simulink subsystem "NIBP_NoiseRemovalFilter_SR"  (R2021b)
settings: Solver=VariableStepAuto  StartTime=0.0  StopTime=10.0  RelTol=1e-3
libraries: Heart_Signal_Processing_Library x5
settings Model: Creator=wallyproenza  LastModifiedBy=wallyproenza

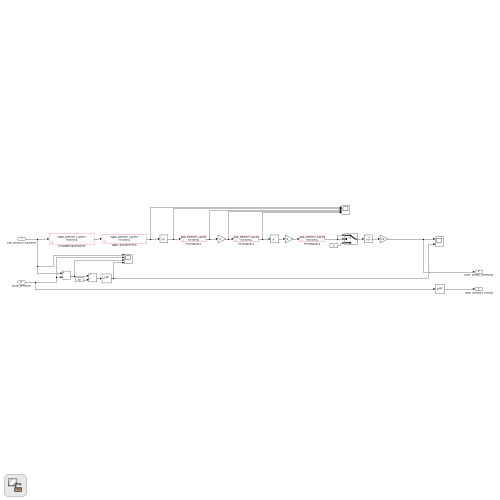
[thumbnail: Simulink's stored preview of the top-level diagram]
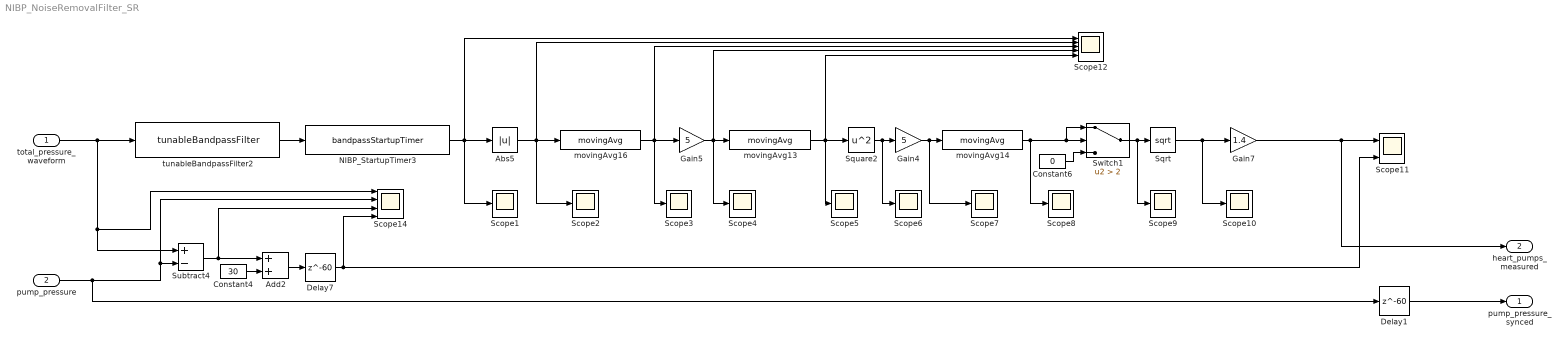
== system NIBP_NoiseRemovalFilter_SR ==
  total_pressure_waveform : Inport
  pump_pressure : Inport  Port=2
  Abs5 : Abs
  Add2 : Sum
  Constant4 : Constant  Value=30
  Constant6 : Constant  Value=0
  Delay1 : Delay  DelayLength=60  InitialCondition=0
  Delay7 : Delay  DelayLength=60  InitialCondition=0
  Gain4 : Gain  Gain=5
  Gain5 : Gain  Gain=5
  Gain7 : Gain  Gain=1.4
  NIBP_StartupTimer3 : Heart_Signal_Processing_Library/bandpassStartupTimer  Description=|  SystemSampleTime=-1  VariantActivationTime=update diagram  Latency=0  AutoFrameSizeCalculation=off
      | The bandpassStartupTimer acts as a temporary buffer between the first 0.5 seconds of the chosen bandpass and the derivative filters.
      | Outputs 0 prior to the 0.5 seconds, and then passes the bandpass filter otuput into the derivative filter after the 0.5 seconds. This component 
      | helps eliminate the possiblility of false negatives caused by an abnormally high signal threshold initial values that could occur prior to 0.5 seconds.
  Scope{1..10} (10 alike) : Scope
  Scope11 : Scope  NumInputPorts=2
  Scope12 : Scope  NumInputPorts=5
  Scope14 : Scope  NumInputPorts=4
  Sqrt : Sqrt  SaturateOnIntegerOverflow=on
  Square2 : Math  Operator=square  SaturateOnIntegerOverflow=on
  Subtract4 : Sum  Inputs=+-
  Switch1 : Switch  Criteria=u2 > Threshold  Threshold=2
  movingAvg13 : Heart_Signal_Processing_Library/movingAvg  Description=|  SystemSampleTime=-1  VariantActivationTime=update diagram  Latency=0  AutoFrameSizeCalculation=off
      | The movingAvg (moving average) filter is designed to be placed after a squaring function (which should have been placed right after the derivative filter),
      | and is a done so that the area where the QRS is present is expanded in regards to timespan. 
      | 
      | The moving average filter takes the average of the most recent 38 samples. This is implemented with a running sum of the most recent 38 samples 
      | with the 39th oldest sample subtracted whenever a new sample is introduced to the sum. Then the sum is divided by 38.
  movingAvg14 : Heart_Signal_Processing_Library/movingAvg  Description=|  SystemSampleTime=-1  VariantActivationTime=update diagram  Latency=0  AutoFrameSizeCalculation=off
      | The movingAvg (moving average) filter is designed to be placed after a squaring function (which should have been placed right after the derivative filter),
      | and is a done so that the area where the QRS is present is expanded in regards to timespan. 
      | 
      | The moving average filter takes the average of the most recent 38 samples. This is implemented with a running sum of the most recent 38 samples 
      | with the 39th oldest sample subtracted whenever a new sample is introduced to the sum. Then the sum is divided by 38.
  movingAvg16 : Heart_Signal_Processing_Library/movingAvg  Description=|  SystemSampleTime=-1  VariantActivationTime=update diagram  Latency=0  AutoFrameSizeCalculation=off
      | The movingAvg (moving average) filter is designed to be placed after a squaring function (which should have been placed right after the derivative filter),
      | and is a done so that the area where the QRS is present is expanded in regards to timespan. 
      | 
      | The moving average filter takes the average of the most recent 38 samples. This is implemented with a running sum of the most recent 38 samples 
      | with the 39th oldest sample subtracted whenever a new sample is introduced to the sum. Then the sum is divided by 38.
  tunableBandpassFilter2 : Heart_Signal_Processing_Library/tunableBandpassFilter  Description=|  SystemSampleTime=-1  VariantActivationTime=update diagram  Latency=0  AutoFrameSizeCalculation=off
      | Bandpass Filter described by the following diference equation in terms of tunable centerFrequency f_o and qualityFactor Q:
      | y[n]=1/(250*10^3+π*10^3*f_o/Q  +4π^2 f_o^2 )*(π*10^3*f_o/Q x[n]  − π*10^3*f_o/Q x[n−2]  −(250*10^3−π*10^3*f_o/Q  +4π^2 f_o^2 )y[n−2]−2*(4π^2 f_o^2  −250*10^3 )y[n−1])
      | 
      | 
      | For simplicity, let constants A, B, and C be subsystems that contain the corresponding defintiions of the coefficients:
      | y[n] = 1/(A+ B + C ) * {Bx[n]  − Bx[n−2]  − (A − B + C )y[n−2]− 2*(C  − A)y[n−1]}
      | 
      | where,
      | A = 250*10^3
      | B = π*10^3*f_o/Q  
      | C = 4π^2 f_o^2
  pump_pressure_synced : Outport
  heart_pumps_measured : Outport  Port=2
  wires:
  Delay1/1 -> pump_pressure_synced/1
  Gain4/1 -> movingAvg14/1, Scope7/1
  Delay7/1 -> Scope11/2, Scope14/4
  Gain7/1 -> Scope11/1, heart_pumps_measured/1
  Gain5/1 -> movingAvg13/1, Scope12/4, Scope4/1
  movingAvg13/1 -> Square2/1, Scope12/5, Scope5/1
  Add2/1 -> Delay7/1
  Subtract4/1 -> Add2/1, Scope14/3
  Sqrt/1 -> Gain7/1, Scope10/1
  Constant4/1 -> Add2/2
  Square2/1 -> Gain4/1, Scope6/1
  total_pressure_waveform/1 -> tunableBandpassFilter2/1, Subtract4/1, Scope14/1
  pump_pressure/1 -> Subtract4/2, Scope14/2, Delay1/1
  Constant6/1 -> Switch1/3
  Abs5/1 -> movingAvg16/1, Scope12/2, Scope2/1
  tunableBandpassFilter2/1 -> NIBP_StartupTimer3/1
  NIBP_StartupTimer3/1 -> Scope12/1, Abs5/1, Scope1/1
  Switch1/1 -> Sqrt/1, Scope9/1
  movingAvg16/1 -> Scope12/3, Gain5/1, Scope3/1
  movingAvg14/1 -> Switch1/1, Switch1/2, Scope8/1
